simulink library "LiU_Compressor_Model_Lib"  (R2014b)
settings: Solver=ode45  SolverMode=SingleTasking  StartTime=0.0  StopTime=10.0  RelTol=1e-3
undefined symbols (not defined in the file): ParamComp
settings Model: CovMetricSettings=dwe  CovHtmlReporting=off  CovSaveCumulativeToWorkspaceVar=off  CovSaveSingleToWorkspaceVar=off  CovExternalEMLEnable=on  CovSFcnEnable=on  Creator=xavll26  LastModifiedBy=xavll26

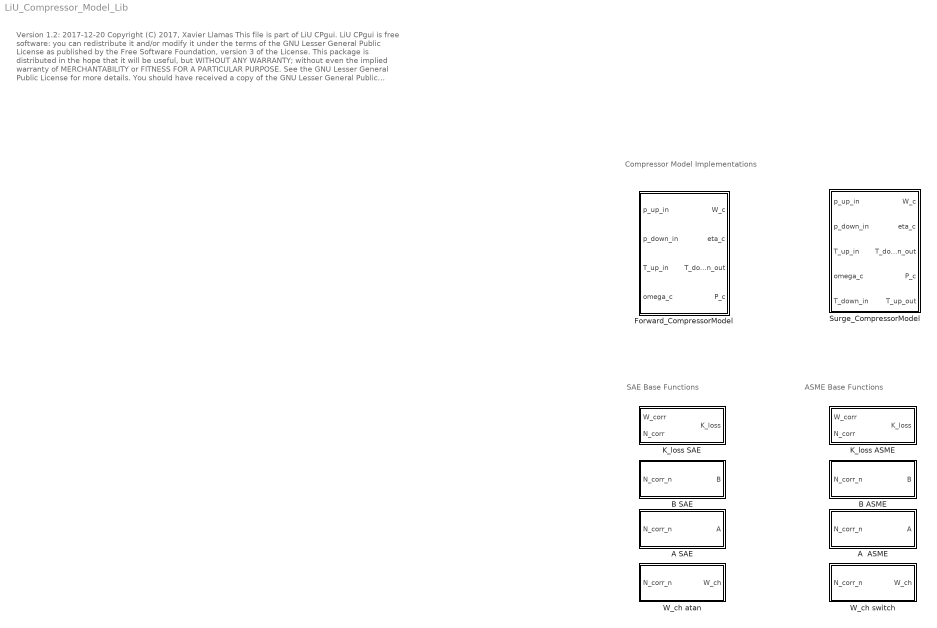
== system LiU_Compressor_Model_Lib ==
  note: Version 1.2: 2017-12-20
      | Copyright (C) 2017, Xavier Llamas
      |
      | This file is part of LiU CPgui.
      | LiU CPgui is free software: you can redistribute it and/or modify
      | it under the terms of the GNU Lesser General Public License as
      | published by the Free Software Foundation, version 3 of the License.
      |
      | This package is distributed in the hope that it will be useful,
      | but WITHOUT ANY WARRANTY; without even the implied warranty of
      | MERCHANTABILITY or FITNESS FOR A PARTICULAR PURPOSE. See the
      | GNU Lesser General Public License for more details.
      |
      | You should have received a copy of the GNU Lesser General Public License
      | along with LiU CPgui. If not, see <http://www.gnu.org/licenses/>.
      |
      | INPUTS
      | p_up_in - Pressure upstream input [Pa]
      | p_down_in - Pressure downstream input [Pa]
      | T_up_in - Temperature upstream input [K]
      | omega_c - Compressor speed [rad/s]
      | T_down_in - Temperature downstream input (when reversed flow) [K]
      | Nc_corr_n - Normalized corrected compressor speed [-]
      | Nc_corr - Corrected compressor speed [rpm]
      | W_corr - Corrected Mass flow [kg/s]
      |
      | OUTPUTS
      | W_c - Compressor mass flow [kg/s]
      | eta_c - Compressor efficiency [-]
      | T_down_out - Temperature downstream output [K]
      | P_c - Compressor power consumed [W]
      | T_up_out - Temperature upstream output (when reversed flow) [K]
      | W_ch - Choke mass flow [kg/s]
      | A - Efficiency A base function [kJ s/kg^2]
      | B - Efficiency B base function [kJ/kg]
      | K_loss - Efficiency K_loss function [-]
      |
      | User Instructions:
      | From the parameters returned by the LiU CPgui tool, simply change its name to ParamComp, e.g. ParamComp = paramT;
      |
      | Depending on the choice of base functions done in the tool LiU CPgui during the parameterization, the compressor model simulink implementations
      | need to be updated with the correct base function blocks. Copy the desired base function block and substitute them inside the compressor model implementations
      |
      | The surge implementation requires four extra parameters related to the reversed flow model and the pipe control volume dimensions
      | used in the More-Greitzer formulation. e.g
      | ParamComp.K0 = 0.3; (Compressor operating as a turbine flow parameter)
      | ParamComp.Kt = 2; (Compressor operating as a turbine exponent parameter)
      | ParamComp.D_tube = 0.015; (Pipe control volume diameter)
      | ParamComp.L_tube = 0.2; (Pipe control volume length)
      | ParamComp.eta_c_asTurbine = 0.2; (Constant efficiency when flow reverses, compressor operating as a poor turbine)
      |
      | If you found this package useful for your research, please cite our work using one or more of the references below.
      |
      | More information:
      |
      | Llamas, X. and Eriksson, L., LiU CPgui: A Toolbox for Parameterizing Compressor Models, Technical Report Nr. LiTH-ISY-R-3102.
      | Department of Electrical Engineering, Linköping University, SE-581 83 Linköping, Sweden, 2018.
      |
      | Llamas, X. and Eriksson, L., Control-Oriented Compressor Model with Adiabatic Efficiency Extrapolation,
      | SAE Int. J. Engines 10(4):2017, doi:10.4271/2017-01-1032.
      |
      | L lamas, X., and Eriksson, L., Parameterizing Compact and Extensible Compressor Models Using Orthogonal Distance Minimization.
      | ASME. J. Eng. Gas Turbines Power. 2016;139(1):012601-012601-10. doi:10.1115/1.4034152.
      |
      | Eriksson, L. , and Nielsen, L. , 2014, Modeling and Control of Engines and Drivelines, Wiley, Hoboken, NJ.
  note: SAE Base Functions
  note: ASME Base Functions
  note: Compressor Model Implementations
  A  ASME : Subsystem
  A SAE : Subsystem
  B ASME : Subsystem
  B SAE : Subsystem
  Forward_CompressorModel : Subsystem
  K_loss ASME : Subsystem
  K_loss SAE : Subsystem
  Surge_CompressorModel : Subsystem
  W_ch atan : Subsystem
  W_ch switch : Subsystem

== system LiU_Compressor_Model_Lib/A  ASME ==
  N_corr_n : Inport
  A param : Constant  Value=ParamComp.C_a
  Delta_h_max : Constant  Value=ParamComp.Delta_h_max  VectorParams1D=off
  Fcn A : Fcn  Expr=-(u[2]*u[1]-u[3]*u[1]^2)*u(4)/u(5)
  Mux2 : Mux
  Wc_max_map : Constant  Value=ParamComp.Wc_max_map  VectorParams1D=off
  A : Outport
  wires:
  A param/1 -> Mux2/2
  N_corr_n/1 -> Mux2/1
  Delta_h_max/1 -> Mux2/3
  Wc_max_map/1 -> Mux2/4
  Fcn A/1 -> A/1
  Mux2/1 -> Fcn A/1

== system LiU_Compressor_Model_Lib/A SAE ==
  N_corr_n : Inport
  A param : Constant  Value=ParamComp.C_a
  Delta_h_max : Constant  Value=ParamComp.Delta_h_max  VectorParams1D=off
  Fcn A : Fcn  Expr=-(u(5)/u(6))*(u(2)*u(1)/((1+u(3)*u(1)^2)^u(4)))
  Mux2 : Mux
  Wc_max_map : Constant  Value=ParamComp.Wc_max_map  VectorParams1D=off
  A : Outport
  wires:
  Mux2/1 -> Fcn A/1
  A param/1 -> Mux2/2
  N_corr_n/1 -> Mux2/1
  Delta_h_max/1 -> Mux2/3
  Wc_max_map/1 -> Mux2/4
  Fcn A/1 -> A/1

== system LiU_Compressor_Model_Lib/B ASME ==
  N_corr_n : Inport
  B param : Constant  Value=ParamComp.C_b
  Delta_h_max : Constant  Value=ParamComp.Delta_h_max  VectorParams1D=off
  Fcn B : Fcn  Expr=u(4)*(u[2]*u[1]+u[3]*u[1]^2)
  Mux1 : Mux  Inputs=3
  B : Outport
  wires:
  Mux1/1 -> Fcn B/1
  B param/1 -> Mux1/2
  N_corr_n/1 -> Mux1/1
  Fcn B/1 -> B/1  "B"
  Delta_h_max/1 -> Mux1/3

== system LiU_Compressor_Model_Lib/B SAE ==
  N_corr_n : Inport
  B param : Constant  Value=ParamComp.C_b
  Delta_h_max : Constant  Value=ParamComp.Delta_h_max  VectorParams1D=off
  Fcn B : Fcn  Expr=u(4)*(u[2]*u[1]^2+u[3]*u[1]^3)
  Mux1 : Mux  Inputs=3
  B : Outport
  wires:
  Mux1/1 -> Fcn B/1
  B param/1 -> Mux1/2
  N_corr_n/1 -> Mux1/1
  Fcn B/1 -> B/1  "B"
  Delta_h_max/1 -> Mux1/3

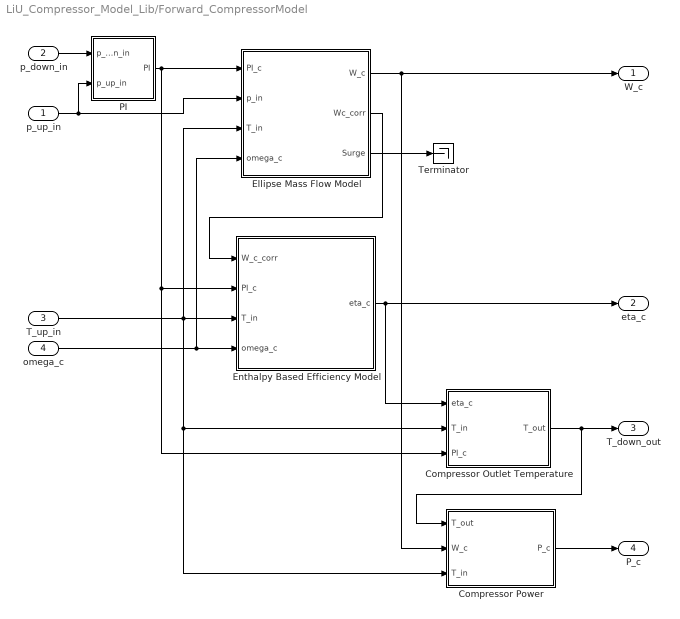
== system LiU_Compressor_Model_Lib/Forward_CompressorModel ==
  p_up_in : Inport
  p_down_in : Inport  Port=2
  T_up_in : Inport  Port=3
  omega_c : Inport  Port=4
  Compressor Outlet Temperature : Subsystem
  Compressor Power : Subsystem
  Ellipse Mass Flow Model : Subsystem
  Enthalpy Based Efficiency Model : Subsystem
  PI : Subsystem
  Terminator : Terminator
  W_c : Outport
  eta_c : Outport  Port=2
  T_down_out : Outport  Port=3
  P_c : Outport  Port=4
  wires:
  omega_c/1 -> Enthalpy Based Efficiency Model/4(omega_c), Ellipse Mass Flow Model/4(omega_c)
  p_up_in/1 -> PI/2(p_up_in), Ellipse Mass Flow Model/2(p_in)
  p_down_in/1 -> PI/1(p_down_in)
  Ellipse Mass Flow Model/1("W_c ") -> Compressor Power/2(W_c), W_c/1
  Enthalpy Based Efficiency Model/1("eta_c ") -> Compressor Outlet Temperature/1(eta_c), eta_c/1
  PI/1(PI) -> Ellipse Mass Flow Model/1(PI_c), Compressor Outlet Temperature/3(PI_c), Enthalpy Based Efficiency Model/2(PI_c)
  Ellipse Mass Flow Model/2("Wc_corr ") -> Enthalpy Based Efficiency Model/1(W_c_corr)
  Ellipse Mass Flow Model/3(Surge) -> Terminator/1
  Compressor Power/1(P_c) -> P_c/1
  Compressor Outlet Temperature/1(T_out) -> Compressor Power/1(T_out), T_down_out/1
  T_up_in/1 -> Compressor Outlet Temperature/2(T_in), Compressor Power/3(T_in), Enthalpy Based Efficiency Model/3(T_in), Ellipse Mass Flow Model/3(T_in)

== system LiU_Compressor_Model_Lib/K_loss ASME ==
  W_corr : Inport
  N_corr : Inport  Port=2
  Constant : Constant
  Terminator : Terminator
  Terminator1 : Terminator
  K_loss : Outport
  wires:
  N_corr/1 -> Terminator/1  "N_corr"
  Constant/1 -> K_loss/1
  W_corr/1 -> Terminator1/1

== system LiU_Compressor_Model_Lib/K_loss SAE ==
  W_corr : Inport
  N_corr : Inport  Port=2
  Fcn K_loss : Fcn  Expr=1+ParamComp.C_loss*(ParamComp.rho1*ParamComp.D_2^3*pi/60)*(u(1)/u(2))
  Mux5 : Mux  Inputs=2
  K_loss : Outport
  wires:
  N_corr/1 -> Mux5/1  "N_corr"
  W_corr/1 -> Mux5/2
  Mux5/1 -> Fcn K_loss/1
  Fcn K_loss/1 -> K_loss/1

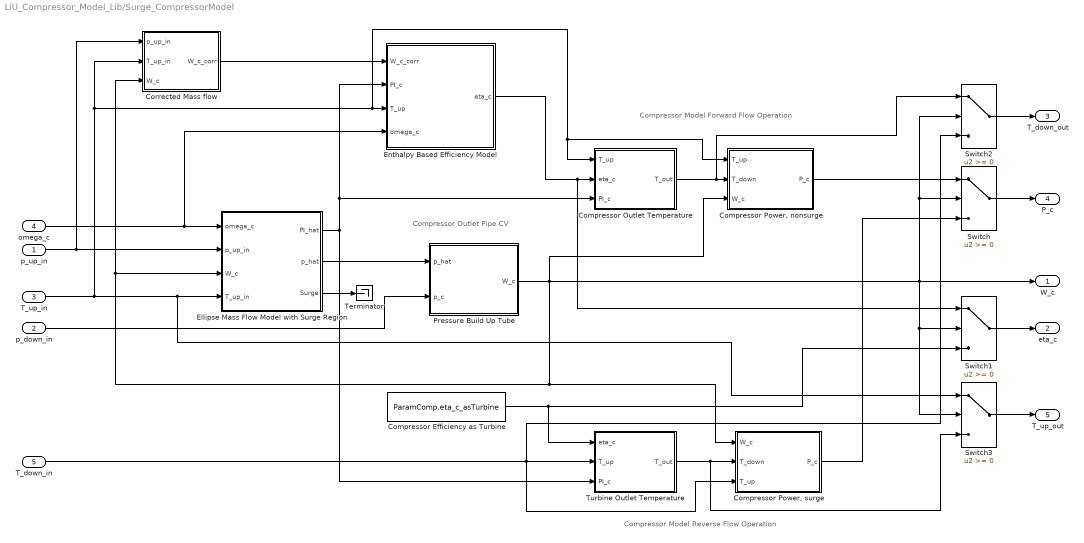
== system LiU_Compressor_Model_Lib/Surge_CompressorModel ==
  note: Compressor Model Forward Flow Operation
  note: Compressor Model Reverse Flow Operation
  note: Compressor Outlet Pipe CV
  p_up_in : Inport
  p_down_in : Inport  Port=2
  T_up_in : Inport  Port=3
  omega_c : Inport  Port=4
  T_down_in : Inport  Port=5
  Compressor Efficiency as Turbine : Constant  Value=ParamComp.eta_c_asTurbine
  Compressor Outlet Temperature : Subsystem
  "Compressor Power, nonsurge" : Subsystem
  "Compressor Power, surge" : Subsystem
  Corrected Mass flow : Subsystem
  Ellipse Mass Flow Model with Surge Region : Subsystem
  Enthalpy Based Efficiency Model : Subsystem
  Pressure Build Up Tube : Subsystem  mask{D=ParamComp.D_tube, L=ParamComp.L_tube}
      mask prompts: D "D. Diameter"; L "L. Length"
  Switch{,1..3} (4 alike) : Switch  ZeroCross=off
  Terminator : Terminator
  Turbine Outlet Temperature : Subsystem
  W_c : Outport
  eta_c : Outport  Port=2
  T_down_out : Outport  Port=3
  P_c : Outport  Port=4
  T_up_out : Outport  Port=5
  wires:
  p_up_in/1 -> Corrected Mass flow/1(p_up_in), Ellipse Mass Flow Model with Surge Region/2(p_up_in)
  p_down_in/1 -> Pressure Build Up Tube/2(p_c)
  Corrected Mass flow/1(W_c_corr) -> Enthalpy Based Efficiency Model/1(W_c_corr)
  omega_c/1 -> Enthalpy Based Efficiency Model/4(omega_c), Ellipse Mass Flow Model with Surge Region/1(omega_c)
  Ellipse Mass Flow Model with Surge Region/2("p_hat ") -> Pressure Build Up Tube/1(p_hat)
  Pressure Build Up Tube/1(W_c) -> Switch2/2, Switch/2, Switch3/2, Switch1/2, W_c/1, "Compressor Power, surge"/1(W_c), Ellipse Mass Flow Model with Surge Region/3(W_c), Corrected Mass flow/3(W_c), "Compressor Power, nonsurge"/3(W_c)
  T_up_in/1 -> Compressor Outlet Temperature/1(T_up), "Compressor Power, nonsurge"/1(T_up), Enthalpy Based Efficiency Model/3(T_up), Corrected Mass flow/2(T_up_in), Switch3/1, Ellipse Mass Flow Model with Surge Region/4(T_up_in)
  Ellipse Mass Flow Model with Surge Region/1("PI_hat ") -> Compressor Outlet Temperature/3(PI_c), Enthalpy Based Efficiency Model/2(PI_c), Turbine Outlet Temperature/3(PI_c)
  Enthalpy Based Efficiency Model/1("eta_c ") -> Switch1/1, Compressor Outlet Temperature/2(eta_c)
  Compressor Outlet Temperature/1(T_out) -> Switch2/1, "Compressor Power, nonsurge"/2(T_down)
  "Compressor Power, nonsurge"/1(P_c) -> Switch/1
  Switch/1 -> P_c/1
  Ellipse Mass Flow Model with Surge Region/3(Surge) -> Terminator/1
  Compressor Efficiency as Turbine/1 -> Turbine Outlet Temperature/1(eta_c), Switch1/3
  T_down_in/1 -> Switch2/3, "Compressor Power, surge"/3(T_up), Turbine Outlet Temperature/2(T_up)
  Turbine Outlet Temperature/1(T_out) -> "Compressor Power, surge"/2(T_down), Switch3/3
  Switch1/1 -> eta_c/1
  "Compressor Power, surge"/1(P_c) -> Switch/3
  Switch3/1 -> T_up_out/1
  Switch2/1 -> T_down_out/1

== system LiU_Compressor_Model_Lib/W_ch atan ==
  N_corr_n : Inport
  Fcn W_ch atan : Fcn  Expr=ParamComp.Wc_max_map*(u[2]+u[3]*atan(u[4]*u[1]-u[5]))
  Mux5 : Mux  Inputs=2
  W_chk_param : Constant  Value=ParamComp.C_Wch
  W_ch : Outport
  wires:
  N_corr_n/1 -> Mux5/1
  Mux5/1 -> Fcn W_ch atan/1
  W_chk_param/1 -> Mux5/2
  Fcn W_ch atan/1 -> W_ch/1

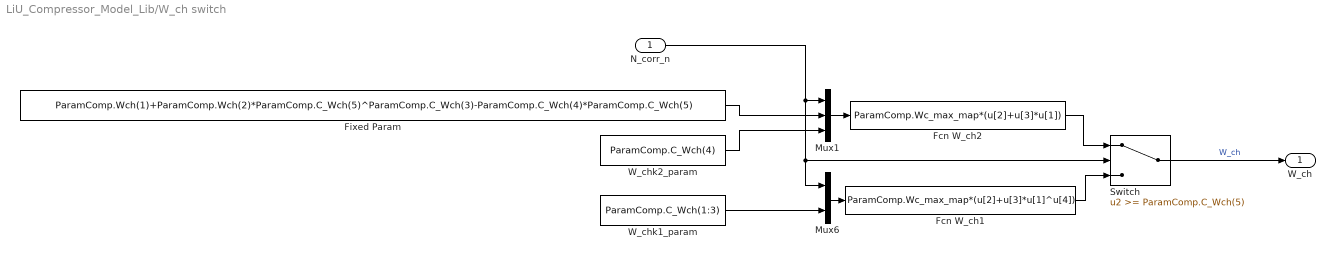
== system LiU_Compressor_Model_Lib/W_ch switch ==
  N_corr_n : Inport
  Fcn W_ch1 : Fcn  Expr=ParamComp.Wc_max_map*(u[2]+u[3]*u[1]^u[4])
  Fcn W_ch2 : Fcn  Expr=ParamComp.Wc_max_map*(u[2]+u[3]*u[1])
  Fixed Param : Constant  Value=ParamComp.Wch(1)+ParamComp.Wch(2)*ParamComp.C_Wch(5)^ParamComp.C_Wch(3)-ParamComp.C_Wch(4)*ParamComp.C_Wch(5)
  Mux1 : Mux  Inputs=3
  Mux6 : Mux  Inputs=2
  Switch : Switch  Threshold=ParamComp.C_Wch(5)
  W_chk1_param : Constant  Value=ParamComp.C_Wch(1:3)
  W_chk2_param : Constant  Value=ParamComp.C_Wch(4)
  W_ch : Outport
  wires:
  N_corr_n/1 -> Mux1/1, Switch/2, Mux6/1
  Mux1/1 -> Fcn W_ch2/1
  Mux6/1 -> Fcn W_ch1/1
  Fcn W_ch2/1 -> Switch/1
  W_chk2_param/1 -> Mux1/3
  W_chk1_param/1 -> Mux6/2
  Fcn W_ch1/1 -> Switch/3
  Switch/1 -> W_ch/1  "W_ch"
  Fixed Param/1 -> Mux1/2

== system LiU_Compressor_Model_Lib/Forward_CompressorModel/Compressor Outlet Temperature ==
  eta_c : Inport
  T_in : Inport  Port=2
  PI_c : Inport  Port=3
  Fcn T_out : Fcn  Expr=u(1)+u(1)/u(3)*(u(2)^((ParamComp.gamma_air - 1)/ParamComp.gamma_air) - 1)
  Mux4 : Mux  Inputs=3
  T_out : Outport
  wires:
  Fcn T_out/1 -> T_out/1
  Mux4/1 -> Fcn T_out/1
  T_in/1 -> Mux4/1
  PI_c/1 -> Mux4/2
  eta_c/1 -> Mux4/3

== system LiU_Compressor_Model_Lib/Forward_CompressorModel/Compressor Power ==
  T_out : Inport
  W_c : Inport  Port=2
  T_in : Inport  Port=3
  Fcn P_c : Fcn  Expr=ParamComp.Cp_air*u(1)*(u(2)-u(3))
  Mux4 : Mux  Inputs=3
  P_c : Outport
  wires:
  Mux4/1 -> Fcn P_c/1
  W_c/1 -> Mux4/1
  T_out/1 -> Mux4/2
  T_in/1 -> Mux4/3
  Fcn P_c/1 -> P_c/1

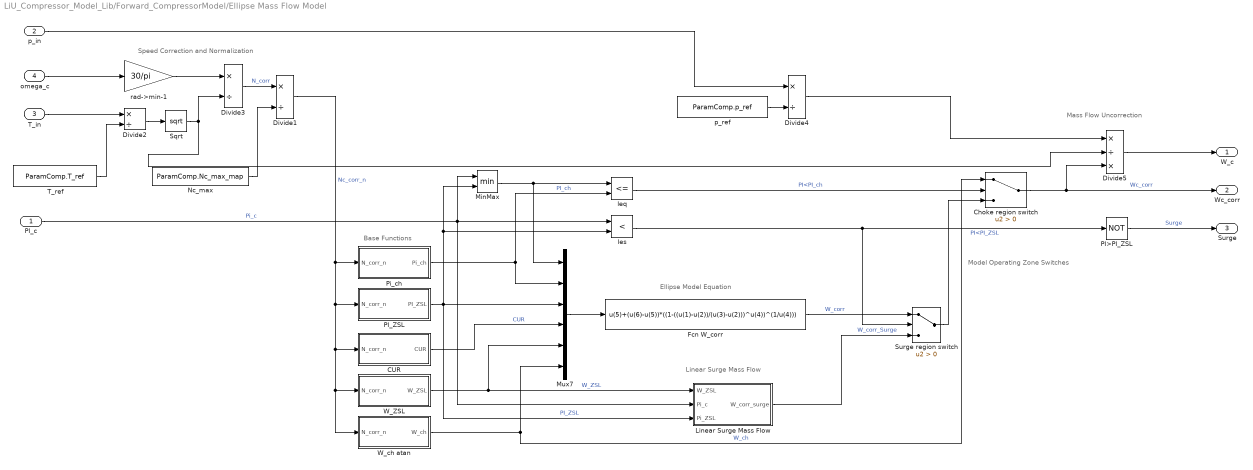
== system LiU_Compressor_Model_Lib/Forward_CompressorModel/Ellipse Mass Flow Model ==
  note: Ellipse Model Equation
  note: Base Functions
  note: Speed Correction and Normalization
  note: Linear Surge Mass Flow
  note: Mass Flow Uncorrection
  note: Model Operating Zone Switches
  PI_c : Inport
  p_in : Inport  Port=2
  T_in : Inport  Port=3
  omega_c : Inport  Port=4
  CUR : Subsystem
  Choke region switch : Switch  Criteria=u2 > Threshold
  Divide{1..4} (4 alike) : Product  Inputs=*/
  Divide5 : Product  Inputs=*/*
  Fcn W_corr : Fcn  Expr=u(5)+(u(6)-u(5))*((1-((u(1)-u(2))/(u(3)-u(2)))^u(4))^(1/u(4)))
  Linear Surge Mass Flow : Subsystem
  MinMax : MinMax  Inputs=2
  Mux7 : Mux  Inputs=6
  Nc_max : Constant  Value=ParamComp.Nc_max_map  VectorParams1D=off
  PI>PI_ZSL : Logic  Operator=NOT  Inputs=1  AllPortsSameDT=off  OutDataTypeStr=boolean
  PI_ZSL : Subsystem
  Pi_ch : Subsystem
  Sqrt : Sqrt  SaturateOnIntegerOverflow=on
  Surge region switch : Switch  Criteria=u2 > Threshold
  T_ref : Constant  Value=ParamComp.T_ref
  W_ZSL : Subsystem
  W_ch atan : Subsystem
  leq : RelationalOperator  Operator=<=  OutDataTypeStr=boolean
  les : RelationalOperator  Operator=<  OutDataTypeStr=boolean
  p_ref : Constant  Value=ParamComp.p_ref
  rad->min-1 : Gain  Gain=30/pi
  "W_c " : Outport
  "Wc_corr " : Outport  Port=2
  Surge : Outport  Port=3
  wires:
  T_in/1 -> Divide2/1
  omega_c/1 -> rad->min-1/1
  rad->min-1/1 -> Divide3/1
  T_ref/1 -> Divide2/2
  Divide2/1 -> Sqrt/1
  Sqrt/1 -> Divide5/2, Divide3/2
  Divide3/1 -> Divide1/1  "N_corr"
  Nc_max/1 -> Divide1/2
  Divide1/1 -> Pi_ch/1(N_corr_n), PI_ZSL/1(N_corr_n), CUR/1(N_corr_n), W_ZSL/1(N_corr_n), W_ch atan/1(N_corr_n)  "Nc_corr_n"
  Mux7/1 -> Fcn W_corr/1
  W_ch atan/1(W_ch) -> Choke region switch/1, Mux7/6  "W_ch"
  W_ZSL/1(W_ZSL) -> Mux7/5, Linear Surge Mass Flow/1(W_ZSL)  "W_ZSL"
  CUR/1(CUR) -> Mux7/4  "CUR"
  Pi_ch/1(Pi_ch) -> Mux7/2, leq/2  "PI_ch"
  PI_c/1 -> MinMax/1, Linear Surge Mass Flow/2(Pi_c), les/1  "Pi_c"
  p_ref/1 -> Divide4/2
  p_in/1 -> Divide4/1
  Divide5/1 -> "W_c "/1
  Divide4/1 -> Divide5/1
  Fcn W_corr/1 -> Surge region switch/1  "W_corr"
  leq/1 -> Choke region switch/2  "PI<PI_ch"
  MinMax/1 -> Mux7/1, leq/1
  Choke region switch/1 -> Divide5/3, "Wc_corr "/1  "Wc_corr"
  PI_ZSL/1(PI_ZSL) -> Linear Surge Mass Flow/3(Pi_ZSL), Mux7/3, les/2, MinMax/2  "PI_ZSL"
  Linear Surge Mass Flow/1(W_corr_surge) -> Surge region switch/3  "W_corr_Surge"
  les/1 -> Surge region switch/2, PI>PI_ZSL/1  "PI<PI_ZSL"
  PI>PI_ZSL/1 -> Surge/1  "Surge"
  Surge region switch/1 -> Choke region switch/3

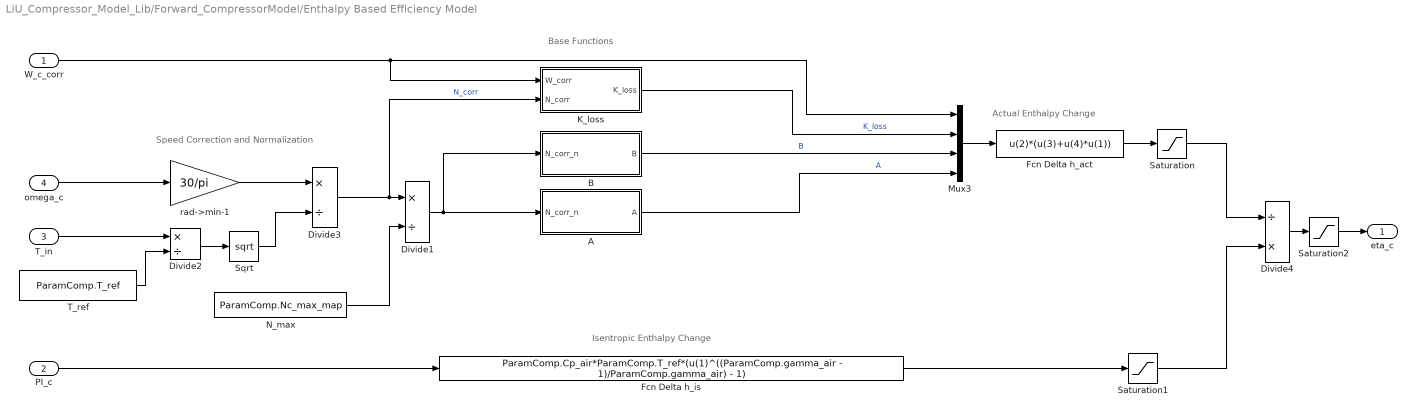
== system LiU_Compressor_Model_Lib/Forward_CompressorModel/Enthalpy Based Efficiency Model ==
  note: Speed Correction and Normalization
  note: Base Functions
  note: Actual Enthalpy Change
  note: Isentropic Enthalpy Change
  W_c_corr : Inport
  PI_c : Inport  Port=2
  T_in : Inport  Port=3
  omega_c : Inport  Port=4
  A : Subsystem
  B : Subsystem
  Divide1 : Product  Inputs=*/
  Divide2 : Product  Inputs=*/
  Divide3 : Product  Inputs=*/
  Divide4 : Product  Inputs=/*
  Fcn Delta h_act : Fcn  Expr=u(2)*(u(3)+u(4)*u(1))
  Fcn Delta h_is : Fcn  Expr=ParamComp.Cp_air*ParamComp.T_ref*(u(1)^((ParamComp.gamma_air - 1)/ParamComp.gamma_air) - 1)
  K_loss : Subsystem
  Mux3 : Mux
  N_max : Constant  Value=ParamComp.Nc_max_map
  Saturation : Saturate  UpperLimit=inf  LowerLimit=1e-4
  Saturation1 : Saturate  UpperLimit=inf  LowerLimit=1e-4
  Saturation2 : Saturate  UpperLimit=1  LowerLimit=1e-3
  Sqrt : Sqrt  SaturateOnIntegerOverflow=on
  T_ref : Constant  Value=ParamComp.T_ref
  rad->min-1 : Gain  Gain=30/pi
  "eta_c " : Outport
  wires:
  T_in/1 -> Divide2/1
  omega_c/1 -> rad->min-1/1
  rad->min-1/1 -> Divide3/1
  T_ref/1 -> Divide2/2
  Divide2/1 -> Sqrt/1
  Sqrt/1 -> Divide3/2
  Divide3/1 -> K_loss/2(N_corr), Divide1/1  "N_corr"
  N_max/1 -> Divide1/2
  Divide1/1 -> B/1(N_corr_n), A/1(N_corr_n)
  A/1(A) -> Mux3/4  "A"
  B/1(B) -> Mux3/3  "B"
  W_c_corr/1 -> Mux3/1, K_loss/1(W_corr)
  Mux3/1 -> Fcn Delta h_act/1
  Fcn Delta h_act/1 -> Saturation/1
  Saturation/1 -> Divide4/1
  Saturation1/1 -> Divide4/2
  Divide4/1 -> Saturation2/1
  Saturation2/1 -> "eta_c "/1
  PI_c/1 -> Fcn Delta h_is/1
  Fcn Delta h_is/1 -> Saturation1/1
  K_loss/1(K_loss) -> Mux3/2  "K_loss"

== system LiU_Compressor_Model_Lib/Forward_CompressorModel/PI ==
  p_down_in : Inport
  p_up_in : Inport  Port=2
  Product : Product  Inputs=/*  SaturateOnIntegerOverflow=on  OutDataTypeStr=Inherit: Same as first input
  PI : Outport
  wires:
  Product/1 -> PI/1
  p_down_in/1 -> Product/2
  p_up_in/1 -> Product/1

== system LiU_Compressor_Model_Lib/Surge_CompressorModel/Compressor Outlet Temperature ==
  T_up : Inport
  eta_c : Inport  Port=2
  PI_c : Inport  Port=3
  "Fcn T_out, compressor" : Fcn  Expr=u(1)+u(1)/u(3)*(u(2)^((ParamComp.gamma_air - 1)/ParamComp.gamma_air) - 1)
  Mux4 : Mux  Inputs=3
  T_out : Outport
  wires:
  "Fcn T_out, compressor"/1 -> T_out/1
  Mux4/1 -> "Fcn T_out, compressor"/1
  T_up/1 -> Mux4/1
  PI_c/1 -> Mux4/2
  eta_c/1 -> Mux4/3

== system LiU_Compressor_Model_Lib/Surge_CompressorModel/Compressor Power, nonsurge ==
  T_up : Inport
  T_down : Inport  Port=2
  W_c : Inport  Port=3
  Fcn P_c : Fcn  Expr=ParamComp.Cp_air*u(1)*(u(2)-u(3))
  Mux4 : Mux  Inputs=3
  P_c : Outport
  wires:
  Mux4/1 -> Fcn P_c/1
  W_c/1 -> Mux4/1
  T_down/1 -> Mux4/2
  T_up/1 -> Mux4/3
  Fcn P_c/1 -> P_c/1

== system LiU_Compressor_Model_Lib/Surge_CompressorModel/Compressor Power, surge ==
  W_c : Inport
  T_down : Inport  Port=2
  T_up : Inport  Port=3
  Fcn P_c : Fcn  Expr=ParamComp.Cp_air*u(1)*(u(3)-u(2))
  Mux4 : Mux  Inputs=3
  P_c : Outport
  wires:
  Mux4/1 -> Fcn P_c/1
  W_c/1 -> Mux4/1
  T_down/1 -> Mux4/2
  T_up/1 -> Mux4/3
  Fcn P_c/1 -> P_c/1

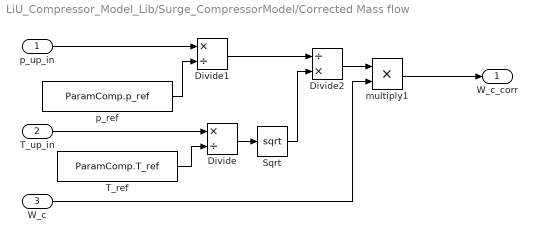
== system LiU_Compressor_Model_Lib/Surge_CompressorModel/Corrected Mass flow ==
  p_up_in : Inport
  T_up_in : Inport  Port=2
  W_c : Inport  Port=3
  Divide : Product  Inputs=*/
  Divide1 : Product  Inputs=*/
  Divide2 : Product  Inputs=/*
  Sqrt : Sqrt  SaturateOnIntegerOverflow=on
  T_ref : Constant  Value=ParamComp.T_ref
  multiply1 : Product  RndMeth=Zero
  p_ref : Constant  Value=ParamComp.p_ref
  W_c_corr : Outport
  wires:
  W_c/1 -> multiply1/2
  Divide2/1 -> multiply1/1
  Divide1/1 -> Divide2/1
  Sqrt/1 -> Divide2/2
  p_up_in/1 -> Divide1/1
  p_ref/1 -> Divide1/2
  Divide/1 -> Sqrt/1
  T_up_in/1 -> Divide/1
  T_ref/1 -> Divide/2
  multiply1/1 -> W_c_corr/1

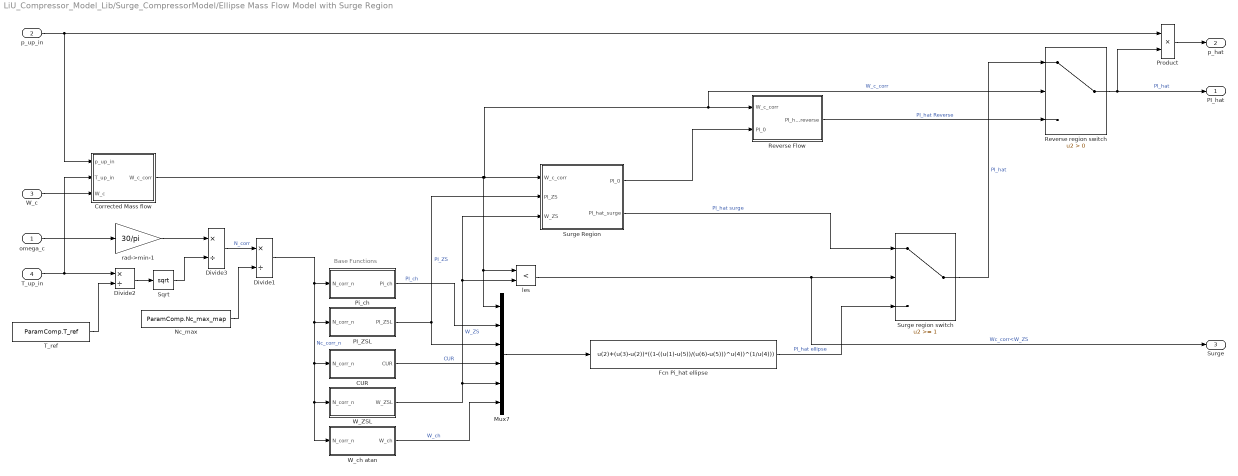
== system LiU_Compressor_Model_Lib/Surge_CompressorModel/Ellipse Mass Flow Model with Surge Region ==
  note: Base Functions
  omega_c : Inport
  p_up_in : Inport  Port=2
  W_c : Inport  Port=3
  T_up_in : Inport  Port=4
  CUR : Subsystem
  Corrected Mass flow : Subsystem
  Divide1 : Product  Inputs=*/
  Divide2 : Product  Inputs=*/
  Divide3 : Product  Inputs=*/
  Fcn Pi_hat ellipse : Fcn  Expr=u(2)+(u(3)-u(2))*((1-((u(1)-u(5))/(u(6)-u(5)))^u(4))^(1/u(4)))
  Mux7 : Mux  Inputs=6
  Nc_max : Constant  Value=ParamComp.Nc_max_map  VectorParams1D=off
  PI_ZSL : Subsystem
  Pi_ch : Subsystem
  Product : Product  Inputs=**  SaturateOnIntegerOverflow=on  OutDataTypeStr=Inherit: Same as first input
  Reverse Flow : Subsystem
  Reverse region switch : Switch  Criteria=u2 > Threshold
  Sqrt : Sqrt  SaturateOnIntegerOverflow=on
  Surge Region : Subsystem
  Surge region switch : Switch  Threshold=1
  T_ref : Constant  Value=ParamComp.T_ref
  W_ZSL : Subsystem
  W_ch atan : Subsystem
  les : RelationalOperator  Operator=<  OutDataTypeStr=boolean
  rad->min-1 : Gain  Gain=30/pi
  "PI_hat " : Outport
  "p_hat " : Outport  Port=2
  Surge : Outport  Port=3
  wires:
  T_up_in/1 -> Corrected Mass flow/2(T_up_in), Divide2/1
  omega_c/1 -> rad->min-1/1
  rad->min-1/1 -> Divide3/1
  T_ref/1 -> Divide2/2
  Divide2/1 -> Sqrt/1
  Sqrt/1 -> Divide3/2
  Divide3/1 -> Divide1/1  "N_corr"
  Nc_max/1 -> Divide1/2
  Mux7/1 -> Fcn Pi_hat ellipse/1
  W_ch atan/1(W_ch) -> Mux7/6  "W_ch"
  W_ZSL/1(W_ZSL) -> Mux7/5, les/2, Surge Region/3(W_ZS)  "W_ZS"
  CUR/1(CUR) -> Mux7/4  "CUR"
  Pi_ch/1(Pi_ch) -> Mux7/2  "PI_ch"
  p_up_in/1 -> Corrected Mass flow/1(p_up_in), Product/1
  Fcn Pi_hat ellipse/1 -> Surge region switch/3  "PI_hat ellipse"
  PI_ZSL/1(PI_ZSL) -> Surge Region/2(PI_ZS), Mux7/3  "PI_ZS"
  Reverse region switch/1 -> Product/2, "PI_hat "/1  "PI_hat"
  W_c/1 -> Corrected Mass flow/3(W_c)
  Corrected Mass flow/1(W_c_corr) -> Reverse region switch/2, Reverse Flow/1(W_c_corr), Surge Region/1(W_c_corr), les/1, Mux7/1  "W_c_corr"
  les/1 -> Surge region switch/2, Surge/1  "Wc_corr<W_ZS"
  Surge Region/2(PI_hat_surge) -> Surge region switch/1  "PI_hat surge"
  Product/1 -> "p_hat "/1
  Divide1/1 -> W_ch atan/1(N_corr_n), W_ZSL/1(N_corr_n), CUR/1(N_corr_n), PI_ZSL/1(N_corr_n), Pi_ch/1(N_corr_n)  "Nc_corr_n"
  Reverse Flow/1(PI_hat_reverse) -> Reverse region switch/3  "PI_hat Reverse"
  Surge region switch/1 -> Reverse region switch/1  "PI_hat"
  Surge Region/1(PI_0) -> Reverse Flow/2(PI_0)

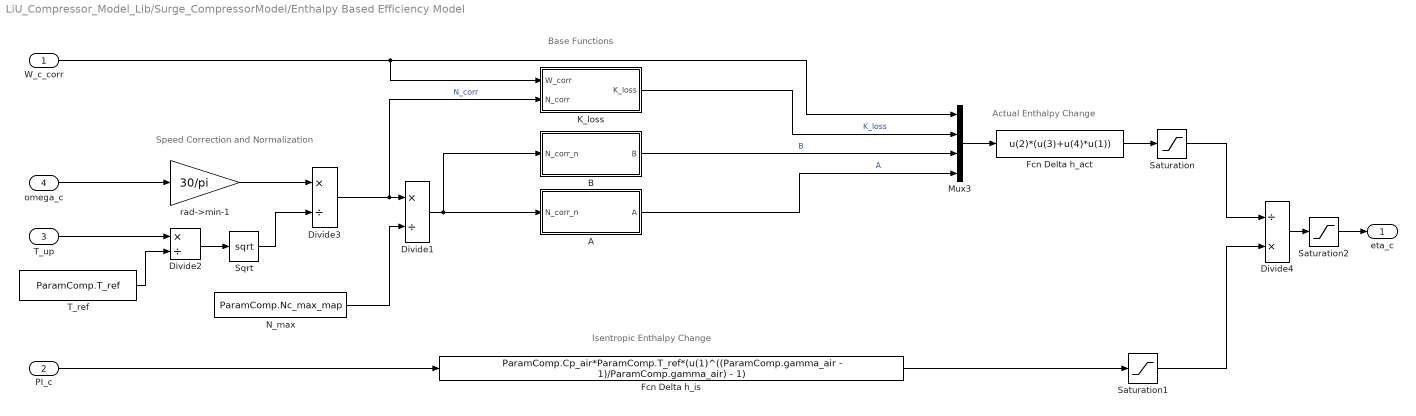
== system LiU_Compressor_Model_Lib/Surge_CompressorModel/Enthalpy Based Efficiency Model ==
  note: Speed Correction and Normalization
  note: Base Functions
  note: Actual Enthalpy Change
  note: Isentropic Enthalpy Change
  W_c_corr : Inport
  PI_c : Inport  Port=2
  T_up : Inport  Port=3
  omega_c : Inport  Port=4
  A : Subsystem
  B : Subsystem
  Divide1 : Product  Inputs=*/
  Divide2 : Product  Inputs=*/
  Divide3 : Product  Inputs=*/
  Divide4 : Product  Inputs=/*
  Fcn Delta h_act : Fcn  Expr=u(2)*(u(3)+u(4)*u(1))
  Fcn Delta h_is : Fcn  Expr=ParamComp.Cp_air*ParamComp.T_ref*(u(1)^((ParamComp.gamma_air - 1)/ParamComp.gamma_air) - 1)
  K_loss : Subsystem
  Mux3 : Mux
  N_max : Constant  Value=ParamComp.Nc_max_map
  Saturation : Saturate  UpperLimit=inf  LowerLimit=1e-4
  Saturation1 : Saturate  UpperLimit=inf  LowerLimit=1e-4
  Saturation2 : Saturate  UpperLimit=1  LowerLimit=1e-3
  Sqrt : Sqrt  SaturateOnIntegerOverflow=on
  T_ref : Constant  Value=ParamComp.T_ref
  rad->min-1 : Gain  Gain=30/pi
  "eta_c " : Outport
  wires:
  T_up/1 -> Divide2/1
  omega_c/1 -> rad->min-1/1
  rad->min-1/1 -> Divide3/1
  T_ref/1 -> Divide2/2
  Divide2/1 -> Sqrt/1
  Sqrt/1 -> Divide3/2
  Divide3/1 -> K_loss/2(N_corr), Divide1/1  "N_corr"
  N_max/1 -> Divide1/2
  Divide1/1 -> B/1(N_corr_n), A/1(N_corr_n)
  A/1(A) -> Mux3/4  "A"
  B/1(B) -> Mux3/3  "B"
  W_c_corr/1 -> Mux3/1, K_loss/1(W_corr)
  Mux3/1 -> Fcn Delta h_act/1
  Fcn Delta h_act/1 -> Saturation/1
  Saturation/1 -> Divide4/1
  Saturation1/1 -> Divide4/2
  Divide4/1 -> Saturation2/1
  Saturation2/1 -> "eta_c "/1
  PI_c/1 -> Fcn Delta h_is/1
  Fcn Delta h_is/1 -> Saturation1/1
  K_loss/1(K_loss) -> Mux3/2  "K_loss"

== system LiU_Compressor_Model_Lib/Surge_CompressorModel/Pressure Build Up Tube ==
  p_hat : Inport
  p_c : Inport  Port=2
  Integrator : Integrator  InitialCondition=0.06  LowerSaturationLimit=0
  add : Sum  Inputs=+-
  pi*D^2/4 : Gain  Gain=(pi*D^2)/(4*L)
  W_c : Outport
  wires:
  pi*D^2/4/1 -> Integrator/1
  add/1 -> pi*D^2/4/1
  p_c/1 -> add/2
  p_hat/1 -> add/1
  Integrator/1 -> W_c/1

== system LiU_Compressor_Model_Lib/Surge_CompressorModel/Turbine Outlet Temperature ==
  eta_c : Inport
  T_up : Inport  Port=2
  PI_c : Inport  Port=3
  "Fcn T_out, turbine" : Fcn  Expr=u(1)-u(1)*u(3)*(1-u(2)^((ParamComp.gamma_air - 1)/ParamComp.gamma_air) )
  Mux4 : Mux  Inputs=3
  T_out : Outport
  wires:
  "Fcn T_out, turbine"/1 -> T_out/1
  Mux4/1 -> "Fcn T_out, turbine"/1
  T_up/1 -> Mux4/1
  PI_c/1 -> Mux4/2
  eta_c/1 -> Mux4/3

== system LiU_Compressor_Model_Lib/Forward_CompressorModel/Ellipse Mass Flow Model/CUR ==
  N_corr_n : Inport
  CUR_param : Constant  Value=ParamComp.C_cur
  Fcn CUR : Fcn  Expr=u[2]+u[3]*u[1]^u[4]
  Mux3 : Mux  Inputs=2
  CUR : Outport
  wires:
  Mux3/1 -> Fcn CUR/1
  CUR_param/1 -> Mux3/2
  N_corr_n/1 -> Mux3/1
  Fcn CUR/1 -> CUR/1

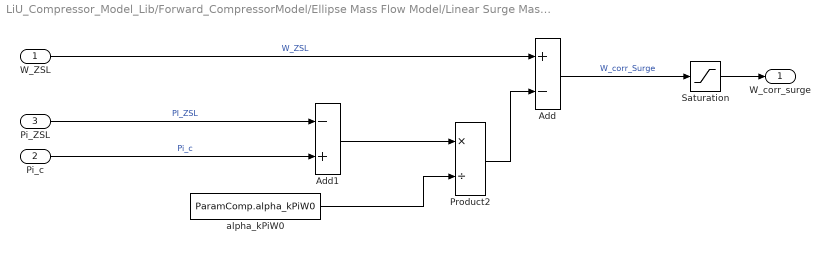
== system LiU_Compressor_Model_Lib/Forward_CompressorModel/Ellipse Mass Flow Model/Linear Surge Mass Flow ==
  W_ZSL : Inport
  Pi_c : Inport  Port=2
  Pi_ZSL : Inport  Port=3
  Add : Sum  Inputs=+-
  Add1 : Sum  Inputs=-+
  Product2 : Product  Inputs=*/
  Saturation : Saturate  UpperLimit=inf  LowerLimit=1e-4
  alpha_kPiW0 : Constant  Value=ParamComp.alpha_kPiW0
  W_corr_surge : Outport
  wires:
  Pi_c/1 -> Add1/2  "Pi_c"
  Pi_ZSL/1 -> Add1/1  "PI_ZSL"
  Add/1 -> Saturation/1  "W_corr_Surge"
  W_ZSL/1 -> Add/1  "W_ZSL"
  Add1/1 -> Product2/1
  alpha_kPiW0/1 -> Product2/2
  Product2/1 -> Add/2
  Saturation/1 -> W_corr_surge/1

== system LiU_Compressor_Model_Lib/Forward_CompressorModel/Ellipse Mass Flow Model/PI_ZSL ==
  N_corr_n : Inport
  Fcn PI_ZSL : Fcn  Expr=1+(ParamComp.PI_max_map-1)*(u[2]*u[1]^u[3])
  Mux2 : Mux  Inputs=2
  Pi_ZSL_param : Constant  Value=ParamComp.C_PIzs
  PI_ZSL : Outport
  wires:
  Mux2/1 -> Fcn PI_ZSL/1
  Pi_ZSL_param/1 -> Mux2/2
  N_corr_n/1 -> Mux2/1
  Fcn PI_ZSL/1 -> PI_ZSL/1

== system LiU_Compressor_Model_Lib/Forward_CompressorModel/Ellipse Mass Flow Model/Pi_ch ==
  N_corr_n : Inport
  Fcn PI_ch : Fcn  Expr=ParamComp.PI_max_map*(u[2]+u[3]*u[1]^u[4])
  Mux1 : Mux  Inputs=2
  Pi_chk_param : Constant  Value=ParamComp.C_PIch
  Pi_ch : Outport
  wires:
  Mux1/1 -> Fcn PI_ch/1
  Pi_chk_param/1 -> Mux1/2
  N_corr_n/1 -> Mux1/1
  Fcn PI_ch/1 -> Pi_ch/1

== system LiU_Compressor_Model_Lib/Forward_CompressorModel/Ellipse Mass Flow Model/W_ZSL ==
  N_corr_n : Inport
  Fcn W_ZSL : Fcn  Expr=ParamComp.Wc_max_map*(u[2]*u[1]^u[3])
  Mux4 : Mux  Inputs=2
  W_ZSL_param : Constant  Value=ParamComp.C_Wzs
  W_ZSL : Outport
  wires:
  Mux4/1 -> Fcn W_ZSL/1
  W_ZSL_param/1 -> Mux4/2
  Fcn W_ZSL/1 -> W_ZSL/1  "W_ZSL"
  N_corr_n/1 -> Mux4/1

== system LiU_Compressor_Model_Lib/Forward_CompressorModel/Ellipse Mass Flow Model/W_ch atan ==
  N_corr_n : Inport
  Fcn W_ch atan : Fcn  Expr=ParamComp.Wc_max_map*(u[2]+u[3]*atan(u[4]*u[1]-u[5]))
  Mux5 : Mux  Inputs=2
  W_chk_param : Constant  Value=ParamComp.C_Wch
  W_ch : Outport
  wires:
  N_corr_n/1 -> Mux5/1
  Mux5/1 -> Fcn W_ch atan/1
  W_chk_param/1 -> Mux5/2
  Fcn W_ch atan/1 -> W_ch/1

== system LiU_Compressor_Model_Lib/Forward_CompressorModel/Enthalpy Based Efficiency Model/A ==
  N_corr_n : Inport
  A param : Constant  Value=ParamComp.C_a
  Delta_h_max : Constant  Value=ParamComp.Delta_h_max  VectorParams1D=off
  Fcn A : Fcn  Expr=-(u(5)/u(6))*(u(2)*u(1)/((1+u(3)*u(1)^2)^u(4)))
  Mux2 : Mux
  Wc_max_map : Constant  Value=ParamComp.Wc_max_map  VectorParams1D=off
  A : Outport
  wires:
  Mux2/1 -> Fcn A/1
  A param/1 -> Mux2/2
  N_corr_n/1 -> Mux2/1
  Delta_h_max/1 -> Mux2/3
  Wc_max_map/1 -> Mux2/4
  Fcn A/1 -> A/1

== system LiU_Compressor_Model_Lib/Forward_CompressorModel/Enthalpy Based Efficiency Model/B ==
  N_corr_n : Inport
  B param : Constant  Value=ParamComp.C_b
  Delta_h_max : Constant  Value=ParamComp.Delta_h_max  VectorParams1D=off
  Fcn B : Fcn  Expr=u(4)*(u[2]*u[1]^2+u[3]*u[1]^3)
  Mux1 : Mux  Inputs=3
  B : Outport
  wires:
  Mux1/1 -> Fcn B/1
  B param/1 -> Mux1/2
  N_corr_n/1 -> Mux1/1
  Fcn B/1 -> B/1  "B"
  Delta_h_max/1 -> Mux1/3

== system LiU_Compressor_Model_Lib/Forward_CompressorModel/Enthalpy Based Efficiency Model/K_loss ==
  W_corr : Inport
  N_corr : Inport  Port=2
  Fcn K_loss : Fcn  Expr=1+ParamComp.C_loss*(ParamComp.rho1*ParamComp.D_2^3*pi/60)*(u(1)/u(2))
  Mux5 : Mux  Inputs=2
  K_loss : Outport
  wires:
  N_corr/1 -> Mux5/1  "N_corr"
  W_corr/1 -> Mux5/2
  Mux5/1 -> Fcn K_loss/1
  Fcn K_loss/1 -> K_loss/1

== system LiU_Compressor_Model_Lib/Surge_CompressorModel/Ellipse Mass Flow Model with Surge Region/CUR ==
  N_corr_n : Inport
  CUR_param : Constant  Value=ParamComp.C_cur
  Fcn CUR : Fcn  Expr=u[2]+u[3]*u[1]^u[4]
  Mux3 : Mux  Inputs=2
  CUR : Outport
  wires:
  Mux3/1 -> Fcn CUR/1
  CUR_param/1 -> Mux3/2
  N_corr_n/1 -> Mux3/1
  Fcn CUR/1 -> CUR/1

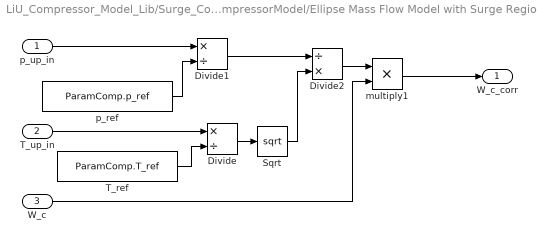
== system LiU_Compressor_Model_Lib/Surge_CompressorModel/Ellipse Mass Flow Model with Surge Region/Corrected Mass flow ==
  p_up_in : Inport
  T_up_in : Inport  Port=2
  W_c : Inport  Port=3
  Divide : Product  Inputs=*/
  Divide1 : Product  Inputs=*/
  Divide2 : Product  Inputs=/*
  Sqrt : Sqrt  SaturateOnIntegerOverflow=on
  T_ref : Constant  Value=ParamComp.T_ref
  multiply1 : Product  RndMeth=Zero
  p_ref : Constant  Value=ParamComp.p_ref
  W_c_corr : Outport
  wires:
  W_c/1 -> multiply1/2
  Divide2/1 -> multiply1/1
  Divide1/1 -> Divide2/1
  Sqrt/1 -> Divide2/2
  p_up_in/1 -> Divide1/1
  p_ref/1 -> Divide1/2
  Divide/1 -> Sqrt/1
  T_up_in/1 -> Divide/1
  T_ref/1 -> Divide/2
  multiply1/1 -> W_c_corr/1

== system LiU_Compressor_Model_Lib/Surge_CompressorModel/Ellipse Mass Flow Model with Surge Region/PI_ZSL ==
  N_corr_n : Inport
  Fcn PI_ZSL : Fcn  Expr=1+(ParamComp.PI_max_map-1)*(u[2]*u[1]^u[3])
  Mux2 : Mux  Inputs=2
  Pi_ZSL_param : Constant  Value=ParamComp.C_PIzs
  PI_ZSL : Outport
  wires:
  Mux2/1 -> Fcn PI_ZSL/1
  Pi_ZSL_param/1 -> Mux2/2
  N_corr_n/1 -> Mux2/1
  Fcn PI_ZSL/1 -> PI_ZSL/1

== system LiU_Compressor_Model_Lib/Surge_CompressorModel/Ellipse Mass Flow Model with Surge Region/Pi_ch ==
  N_corr_n : Inport
  Fcn PI_ch : Fcn  Expr=ParamComp.PI_max_map*(u[2]+u[3]*u[1]^u[4])
  Mux1 : Mux  Inputs=2
  Pi_chk_param : Constant  Value=ParamComp.C_PIch
  Pi_ch : Outport
  wires:
  Mux1/1 -> Fcn PI_ch/1
  Pi_chk_param/1 -> Mux1/2
  N_corr_n/1 -> Mux1/1
  Fcn PI_ch/1 -> Pi_ch/1

== system LiU_Compressor_Model_Lib/Surge_CompressorModel/Ellipse Mass Flow Model with Surge Region/Reverse Flow ==
  W_c_corr : Inport
  PI_0 : Inport  Port=2
  Fcn Pi_hat reverse : Fcn  Expr=-1+u[4]+(1-(-u[3]/(u[1]*ParamComp.Wc_max_map))^2)^(-1/u[2])
  K0 param : Constant  Value=ParamComp.K0
  Kt param : Constant  Value=ParamComp.Kt
  Mux10 : Mux
  PI_hat_reverse : Outport
  wires:
  W_c_corr/1 -> Mux10/3  "W_c_corr"
  PI_0/1 -> Mux10/4  "PI_0"
  Mux10/1 -> Fcn Pi_hat reverse/1
  Kt param/1 -> Mux10/2  "Kt"
  K0 param/1 -> Mux10/1  "K0"
  Fcn Pi_hat reverse/1 -> PI_hat_reverse/1

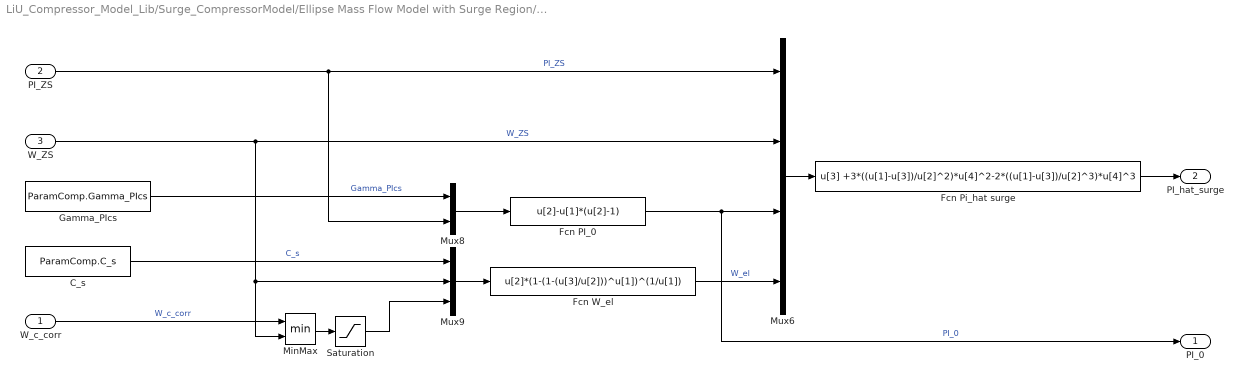
== system LiU_Compressor_Model_Lib/Surge_CompressorModel/Ellipse Mass Flow Model with Surge Region/Surge Region ==
  W_c_corr : Inport
  PI_ZS : Inport  Port=2
  W_ZS : Inport  Port=3
  C_s : Constant  Value=ParamComp.C_s
  Fcn PI_0 : Fcn  Expr=u[2]-u[1]*(u[2]-1)
  Fcn Pi_hat surge : Fcn  Expr=u[3] +3*((u[1]-u[3])/u[2]^2)*u[4]^2-2*((u[1]-u[3])/u[2]^3)*u[4]^3
  Fcn W_el : Fcn  Expr=u[2]*(1-(1-(u[3]/u[2]))^u[1])^(1/u[1])
  Gamma_PIcs : Constant  Value=ParamComp.Gamma_PIcs
  MinMax : MinMax  Inputs=2
  Mux6 : Mux
  Mux8 : Mux  Inputs=2
  Mux9 : Mux  Inputs=3
  Saturation : Saturate  UpperLimit=inf  LowerLimit=0
  PI_0 : Outport
  PI_hat_surge : Outport  Port=2
  wires:
  W_ZS/1 -> Mux6/2, MinMax/2, Mux9/2  "W_ZS"
  PI_ZS/1 -> Mux8/2, Mux6/1  "PI_ZS"
  W_c_corr/1 -> MinMax/1  "W_c_corr"
  Mux6/1 -> Fcn Pi_hat surge/1
  Mux8/1 -> Fcn PI_0/1
  Gamma_PIcs/1 -> Mux8/1  "Gamma_PIcs"
  Mux9/1 -> Fcn W_el/1
  C_s/1 -> Mux9/1  "C_s"
  Fcn W_el/1 -> Mux6/4  "W_el"
  Fcn PI_0/1 -> PI_0/1, Mux6/3  "PI_0"
  MinMax/1 -> Saturation/1
  Saturation/1 -> Mux9/3
  Fcn Pi_hat surge/1 -> PI_hat_surge/1

== system LiU_Compressor_Model_Lib/Surge_CompressorModel/Ellipse Mass Flow Model with Surge Region/W_ZSL ==
  N_corr_n : Inport
  Fcn W_ZSL : Fcn  Expr=ParamComp.Wc_max_map*(u[2]*u[1]^u[3])
  Mux4 : Mux  Inputs=2
  W_ZSL_param : Constant  Value=ParamComp.C_Wzs
  W_ZSL : Outport
  wires:
  Mux4/1 -> Fcn W_ZSL/1
  W_ZSL_param/1 -> Mux4/2
  Fcn W_ZSL/1 -> W_ZSL/1  "W_ZSL"
  N_corr_n/1 -> Mux4/1

== system LiU_Compressor_Model_Lib/Surge_CompressorModel/Ellipse Mass Flow Model with Surge Region/W_ch atan ==
  N_corr_n : Inport
  Fcn W_ch atan : Fcn  Expr=ParamComp.Wc_max_map*(u[2]+u[3]*atan(u[4]*u[1]-u[5]))
  Mux5 : Mux  Inputs=2
  W_chk_param : Constant  Value=ParamComp.C_Wch
  W_ch : Outport
  wires:
  N_corr_n/1 -> Mux5/1
  Mux5/1 -> Fcn W_ch atan/1
  W_chk_param/1 -> Mux5/2
  Fcn W_ch atan/1 -> W_ch/1

== system LiU_Compressor_Model_Lib/Surge_CompressorModel/Enthalpy Based Efficiency Model/A ==
  N_corr_n : Inport
  A param : Constant  Value=ParamComp.C_a
  Delta_h_max : Constant  Value=ParamComp.Delta_h_max  VectorParams1D=off
  Fcn A : Fcn  Expr=-(u(5)/u(6))*(u(2)*u(1)/((1+u(3)*u(1)^2)^u(4)))
  Mux2 : Mux
  Wc_max_map : Constant  Value=ParamComp.Wc_max_map  VectorParams1D=off
  A : Outport
  wires:
  Mux2/1 -> Fcn A/1
  A param/1 -> Mux2/2
  N_corr_n/1 -> Mux2/1
  Delta_h_max/1 -> Mux2/3
  Wc_max_map/1 -> Mux2/4
  Fcn A/1 -> A/1

== system LiU_Compressor_Model_Lib/Surge_CompressorModel/Enthalpy Based Efficiency Model/B ==
  N_corr_n : Inport
  B param : Constant  Value=ParamComp.C_b
  Delta_h_max : Constant  Value=ParamComp.Delta_h_max  VectorParams1D=off
  Fcn B : Fcn  Expr=u(4)*(u[2]*u[1]^2+u[3]*u[1]^3)
  Mux1 : Mux  Inputs=3
  B : Outport
  wires:
  Mux1/1 -> Fcn B/1
  B param/1 -> Mux1/2
  N_corr_n/1 -> Mux1/1
  Fcn B/1 -> B/1  "B"
  Delta_h_max/1 -> Mux1/3

== system LiU_Compressor_Model_Lib/Surge_CompressorModel/Enthalpy Based Efficiency Model/K_loss ==
  W_corr : Inport
  N_corr : Inport  Port=2
  Fcn K_loss : Fcn  Expr=1+ParamComp.C_loss*(ParamComp.rho1*ParamComp.D_2^3*pi/60)*(u(1)/u(2))
  Mux5 : Mux  Inputs=2
  K_loss : Outport
  wires:
  N_corr/1 -> Mux5/1  "N_corr"
  W_corr/1 -> Mux5/2
  Mux5/1 -> Fcn K_loss/1
  Fcn K_loss/1 -> K_loss/1
